simulink model "TestModel"  (R2020b)
settings: Solver=VariableStepAuto  StartTime=0.0  StopTime=inf  RelTol=1e-3
libraries: simulink_extras x2
settings Model: EnablePacing=on  PacingRate=5  Creator=K-110-05  LastModifiedBy=K-110-05

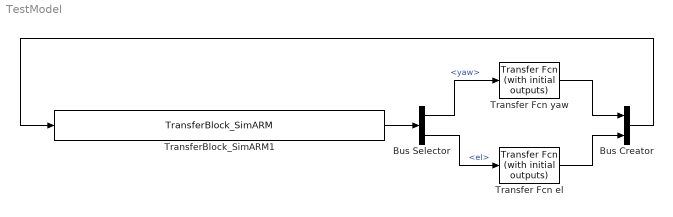
== system TestModel ==
  Bus Creator : BusCreator  Inputs=2  OutDataTypeStr=Bus: AngleData
      settings: InheritFromInputs=off
  Bus Selector : BusSelector  OutputSignals=yaw,el
  Transfer Fcn el : simulink_extras/Additional Linear/Transfer Fcn (with initial outputs)  N=[1]  D="[1  0]"  Y0=90*pi/180  U0=0
  Transfer Fcn yaw : simulink_extras/Additional Linear/Transfer Fcn (with initial outputs)  N=[1]  D="[1  0]"  Y0=0  U0=0
  TransferBlock_SimARM1 : S-Function  FunctionName=TransferBlock_SimARM  SFunctionDeploymentMode=off  EnableBusSupport=off  mask(Legacy Function){SFunctionSpec=void Output_Point_ModelARM(AngleData u1[1], AngleData y1[1]), ShowSpec=on}
      mask prompts: ShowSpec "Display function specification"
      mask help:
      | This block allows you to call the legacy functions specified by the following Legacy Code Tool definition:
      | def.SFunctionName = 'TransferBlock_SimARM';
      | def.OutputFcnSpec = 'void Output_Point_ModelARM(AngleData u1[1], AngleData y1[1])';
      | def.StartFcnSpec = 'void Start_Point_ModelARM()';
      | def.TerminateFcnSpec = 'void Terminate_Point()';
      | def.HeaderFiles = {'Wrapper.hpp', 'SimFederate.hpp'};
      | def.SourceFiles = {'Wrapper.cpp', 'SimFederate.cpp'};
      | def.HostLibFiles = {'HLAlib.lib', 'libfedtime1516e.lib', 'librti1516e.lib', 'rtiexec.lib', 'tbb12.lib'};
      | def.IncPaths = {'C:\QtWork\laboratory\', 'C:\QtWork\laboratory\HLAdata/', 'C:\QtWork\laboratory\HLA-Simulink/SimulinkARM/SimFederate/', 'C:\rrti-2.0\RRTI-2.0.0164\include/HLA2010', 'C:\QtWork\laboratory\3dparty/boost_1_75_0'};
      | def.SrcPaths = {'C:\QtWork\laboratory\', 'C:\QtWork\laboratory\/HLA-Simulink/SimulinkARM/SimFederate/'};
      | def.LibPaths = {'C:\rrti-2.0\RRTI-2.0.0164\bin/', 'C:\QtWork\laboratory\lib/windows/', 'C:\QtWork\laboratory\/3dparty/tbb/lib/intel64/vc14\'};
      mask Help: <p>This block was generated automatically by the Legacy Code Tool. For detailed help on this tool, call<a href="matlab:legacy_code('help')"> legacy_code('help')</a>.</p>
      mask Callback ShowSpec:
      | if strcmp(get_param(gcbh, 'ShowSpec'), 'on')
      |   set_param(gcbh, 'MaskDisplay', sprintf('fprintf(''%s'');', get_param(gcbh, 'SFunctionSpec')));
      | else
      |   set_param(gcbh, 'MaskDisplay', sprintf('fprintf(''%s'');', get_param(gcbh, 'FunctionName')));
      | end
      mask Display: fprintf('void Output_Point_ModelARM(AngleData u1[1], AngleData y1[1])');
  wires:
  TransferBlock_SimARM1/1 -> Bus Selector/1
  Bus Selector/1 -> Transfer Fcn yaw/1  "<yaw>"
  Bus Selector/2 -> Transfer Fcn el/1  "<el>"
  Bus Creator/1 -> TransferBlock_SimARM1/1
  Transfer Fcn yaw/1 -> Bus Creator/1
  Transfer Fcn el/1 -> Bus Creator/2
